simulink subsystem "StateEstimationInterface"  (R2025b)
settings: Solver=VariableStepAuto  StartTime=0.0  StopTime=10.0  RelTol=1e-3
settings Model: Creator=yvijay  LastModifiedBy=YuktiVijay

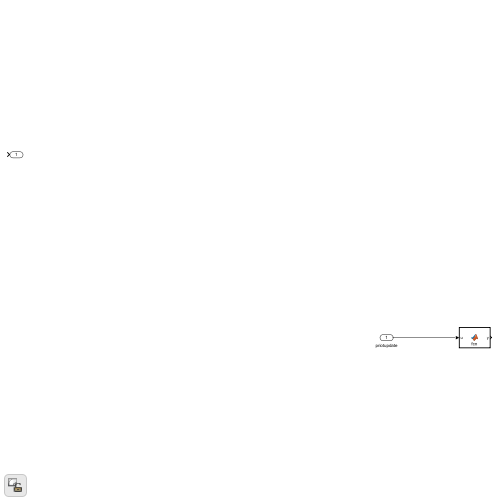
[thumbnail: Simulink's stored preview of the top-level diagram]
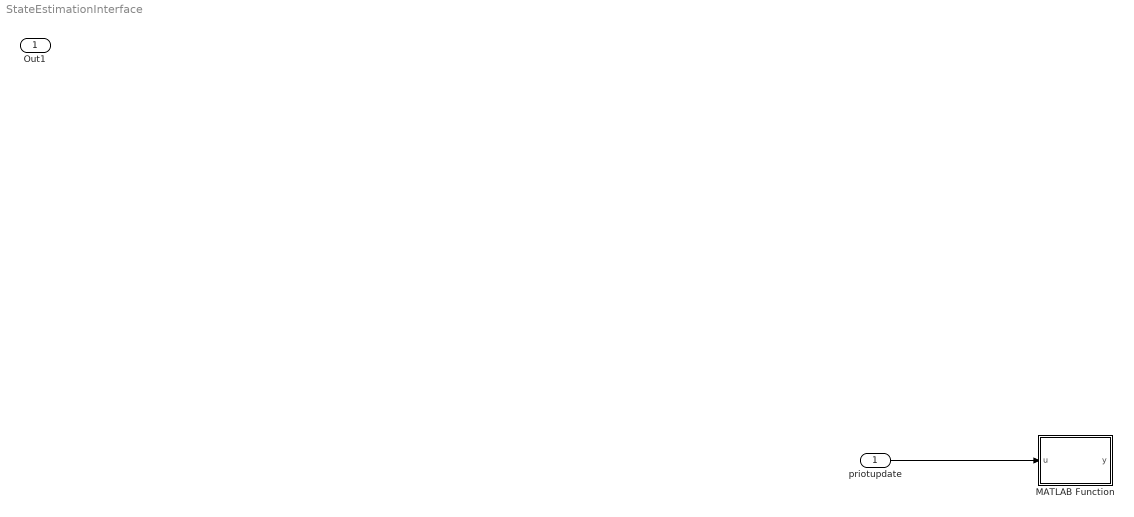
== system StateEstimationInterface ==
  priotupdate : Inport
  MATLAB Function : MATLAB Function  TreatAsAtomicUnit=on
  Out1 : Outport
  wires:
  priotupdate/1 -> MATLAB Function/1(u)

== matlab function StateEstimationInterface/MATLAB Function ==
  data: u input; y output
function y = fcn(u)

y = u;
